simulink library "btg"  (Simulink 8.1)
settings: Solver=ode1  StartTime=0.0  StopTime=Inf  FixedStep=0.001  RelTol=1e-3
PostLoadFcn:
  | , if any(exist('dsrtsu_mdlpostloadfcn', 'file') == [2, 3, 6]), try dsrtsu_mdlpostloadfcn('Execute', bdroot); catch fprintf('Error in PostLoadFcn (dsrtsu_mdlpostloadfcn) for model "%s":\n %s\n', bdroot, lasterr); end, end,
undefined symbols (not defined in the file or in its folder): AACC_VehSpdError_kph, KACC_ACCDefBrakDist_m, KACC_ACCDesDistMarg_m, KACC_BrakeTGapPerc_perc, KACC_ConsideredBrakeSetTimeGap_s, KACC_TransTGapPTBFixedMargin_flg, MACC_ACCLookUpDecelControl_mps2
libraries: hcu_lib x2, simulink x1
settings Model: DSRTSU_INTERNAL_RTI_VER=450  DSRTSU_INTERNAL_RTI_TYPE=rti1401  Creator=AT015555  LastModifiedBy=AT015555

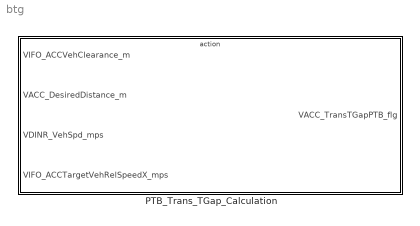
== system btg ==
  PTB_Trans_TGap_Calculation : Subsystem  TreatAsAtomicUnit=on

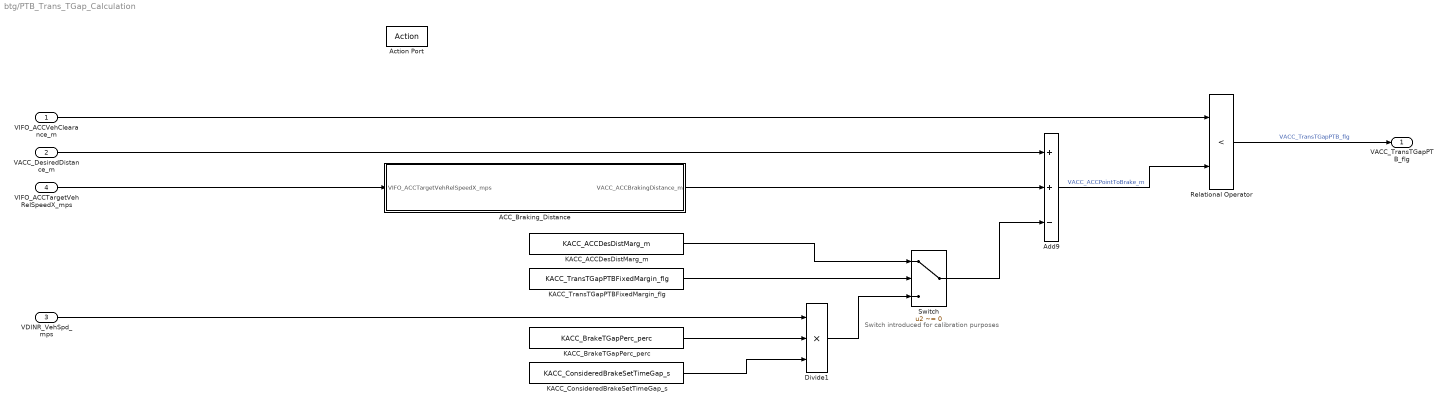
== system btg/PTB_Trans_TGap_Calculation ==
  note: Switch introduced for calibration purposes
  VIFO_ACCVehClearance_m : Inport
  VACC_DesiredDistance_m : Inport  Port=2
  VDINR_VehSpd_mps : Inport  Port=3
  VIFO_ACCTargetVehRelSpeedX_mps : Inport  Port=4
  Action Port : ActionPort
  ACC_Braking_Distance : Subsystem
  Add9 : Sum  Inputs=++-
  Divide1 : Product  Inputs=***
  KACC_ACCDesDistMarg_m : Constant  Value=KACC_ACCDesDistMarg_m
  KACC_BrakeTGapPerc_perc : Constant  Value=KACC_BrakeTGapPerc_perc
  KACC_ConsideredBrakeSetTimeGap_s : Constant  Value=KACC_ConsideredBrakeSetTimeGap_s
  KACC_TransTGapPTBFixedMargin_flg : Constant  Value=KACC_TransTGapPTBFixedMargin_flg
  Relational Operator : RelationalOperator  Operator=<  OutDataTypeStr=boolean
  Switch : Switch  Criteria=u2 ~= 0
  VACC_TransTGapPTB_flg : Outport
  wires:
  Add9/1 -> Relational Operator/2  "VACC_ACCPointToBrake_m"
  VIFO_ACCVehClearance_m/1 -> Relational Operator/1
  VACC_DesiredDistance_m/1 -> Add9/1
  VIFO_ACCTargetVehRelSpeedX_mps/1 -> ACC_Braking_Distance/1(VIFO_ACCTargetVehRelSpeedX_mps)
  ACC_Braking_Distance/1(VACC_ACCBrakingDistance_m) -> Add9/2
  Switch/1 -> Add9/3
  KACC_TransTGapPTBFixedMargin_flg/1 -> Switch/2
  KACC_ConsideredBrakeSetTimeGap_s/1 -> Divide1/3
  KACC_BrakeTGapPerc_perc/1 -> Divide1/2
  VDINR_VehSpd_mps/1 -> Divide1/1
  Divide1/1 -> Switch/3
  KACC_ACCDesDistMarg_m/1 -> Switch/1
  Relational Operator/1 -> VACC_TransTGapPTB_flg/1  "VACC_TransTGapPTB_flg"

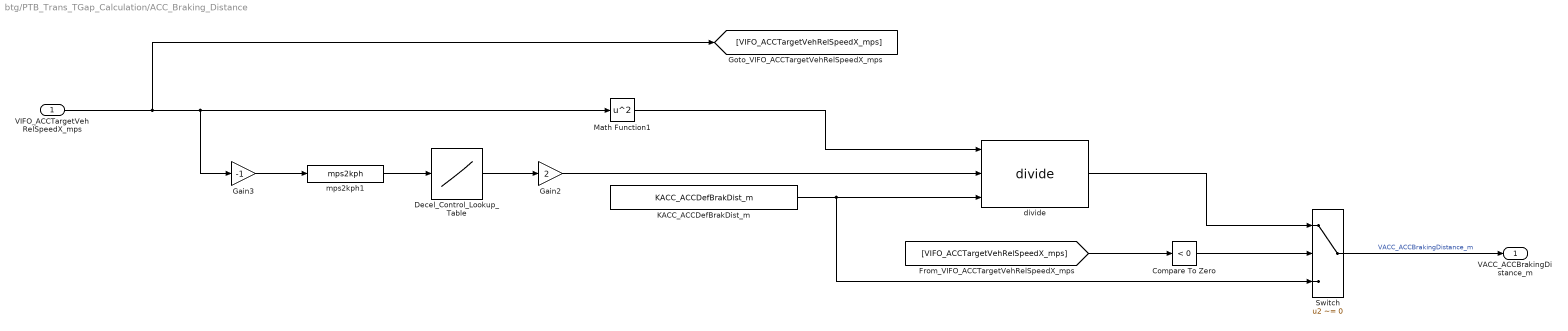
== system btg/PTB_Trans_TGap_Calculation/ACC_Braking_Distance ==
  VIFO_ACCTargetVehRelSpeedX_mps : Inport
  Compare To Zero : simulink/Logic and Bit Operations/Compare To Zero  relop=<  OutDataTypeStr=boolean
  Decel_Control_Lookup_Table : Lookup_n-D  NumberOfTableDimensions=1  BreakpointsForDimension1=AACC_VehSpdError_kph  Table=MACC_ACCLookUpDecelControl_mps2  ExtrapMethod=Clip  UseLastTableValue=on  RndMeth=Simplest  InputSameDT=on
  Gain2 : Gain  Gain=2
  Gain3 : Gain  Gain=-1
  KACC_ACCDefBrakDist_m : Constant  Value=KACC_ACCDefBrakDist_m
  Math Function1 : Math  Operator=square  SaturateOnIntegerOverflow=on
  Switch : Switch  Criteria=u2 ~= 0
  divide : hcu_lib/divide
  mps2kph1 : hcu_lib/mps2kph
  VACC_ACCBrakingDistance_m : Outport
  wires:
  Math Function1/1 -> divide/1
  Switch/1 -> VACC_ACCBrakingDistance_m/1  "VACC_ACCBrakingDistance_m"
  Gain2/1 -> divide/2
  Gain3/1 -> mps2kph1/1
  mps2kph1/1 -> Decel_Control_Lookup_Table/1
  Decel_Control_Lookup_Table/1 -> Gain2/1
  KACC_ACCDefBrakDist_m/1 -> Switch/3, divide/3
  VIFO_ACCTargetVehRelSpeedX_mps/1 -> [VIFO_ACCTargetVehRelSpeedX_mps], Gain3/1, Math Function1/1
  Compare To Zero/1 -> Switch/2
  divide/1 -> Switch/1
  [VIFO_ACCTargetVehRelSpeedX_mps] -> Compare To Zero/1
